simulink model "TestSolidStateTransformer"  (R2025b)
settings: Solver=VariableStepAuto  StartTime=0.0  StopTime=0.5  FixedStep=50e-6  RelTol=1e-3
model workspace (MAT data in the model file):
  sst.chb.Kbal = 0.000227272727273
  sst.dab.kp = 5.5
  sst.dab.ki = 130
  sst.dab.upperLimit = 0.45
  sst.dab.lowerLimit = -0.45
  sst.dab.sampleTime = 5e-05
  sst.dab.Kp_bal = 0.0005
  sst.dab.bal_alpha = 0.998116819821
  ups.sampleTime = 5e-05
undefined symbols (not defined in the file): DiscIntNeverNeededParam, ee_sli_rtmsupport, gcbh, Ts
libraries: fl_lib x23, nesl_utility x20, datacenter_lib x12, ee_lib x9, simulink x8, eeGeneralControl x6, eeTransforms x4, slpidlib x3, eeSinusoidalMeasurementV2 x2, simulink_extras x1
(part 1 of 2)
settings Model: SimulationMode=accelerator  Creator=saprasad  LastModifiedBy=skota
settings SimscapeCC: ExplicitSolverDiagnosticOptions=none

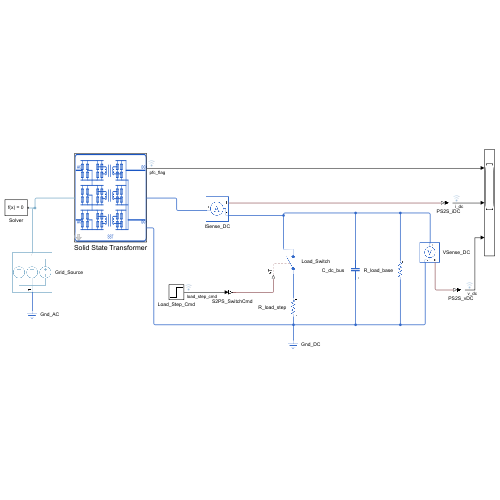
[thumbnail: Simulink's stored preview of the top-level diagram]
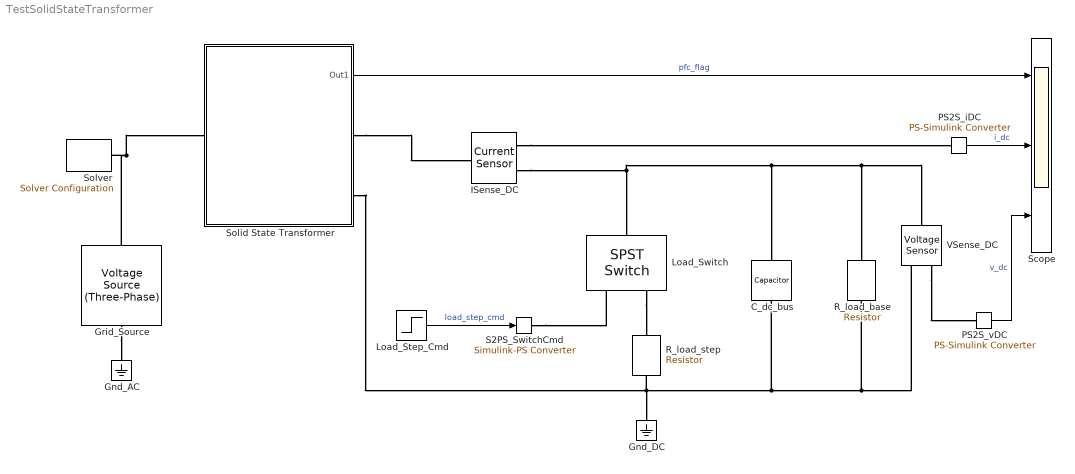
== system TestSolidStateTransformer ==
  C_dc_bus : ee_lib/Passive/Capacitor  cap_option=ee.enum.passive.capacitor.capOption.const  c=20e-3 F  Cvec=[1e-05, 1e-06] F  Vvec=[0, 10] V  CV_table_symmetry=ee.enum.passive.capacitor.tableSymmetry.yes  f_vec=[1, 10] kHz  DFext_vec=[.8, 1.2]  enable_C_tol=ee.enum.toleranceApplication.none  averaging_period=0 s  C_tol=5  tol_distribution=ee.enum.toleranceDistribution.uniform  nSigma=4  r=0 Ohm  g=0 1/Ohm  enable_operating_limits=ee.enum.enable.no  operating_limit_action=ee.enum.passive.reportOpLim.warn  max_working_voltage_range=[-25, 25] V  power_rating=1 W  maxTemperature=85 degC  thermalEnable=false  thermalMass=1 J/K  i_specify=off  i_priority=None  i=0 A  i_nominal_specify=off  i_nominal_value=1  i_nominal_unit=A  v_specify=off  v_priority=None  v=0 V  v_nominal_specify=off  v_nominal_value=1  v_nominal_unit=V  vc_specify=on  vc_priority=None  vc=800 V  vc_nominal_specify=off  vc_nominal_value=1  vc_nominal_unit=V  T_specify=off  T_priority=None  T=298.15 K  T_nominal_specify=off  T_nominal_value=1  T_nominal_unit=K
  Gnd_AC : fl_lib/Electrical/Electrical Elements/Electrical Reference
  Gnd_DC : fl_lib/Electrical/Electrical Elements/Electrical Reference
  Grid_Source : ee_lib/Sources/Voltage Source (Three-Phase)  vline_rms=13800 V  shift=0 deg  freq=60 Hz  impedance_option=1  SShortCircuit=1e9 A*V  XR=15  R=0.01 Ohm  L=3.97e-4 H  harmonic_option=0  harmonic_orders=[5, 7, 11, 13]  harmonic_ratios=[.1, .1, .1, .1]  G_parasitic=0 1/Ohm  I_specify=off  I_priority=None  I=[0, 0, 0] A  I_nominal_specify=off  I_nominal_value=1  I_nominal_unit=A
  ISense_DC : fl_lib/Electrical/Electrical Sensors/Current Sensor
  Load_Step_Cmd : Step  Time=0.3  SampleTime=0
  Load_Switch : ee_lib/Switches & Breakers/SPST Switch  R_closed=1e-3 Ohm  G_open=1e-8 S  Threshold=0.5 V  Width=0 V  model_dynamics=0  t_on=1e-3 s  t_off=1e-3 s  initial_vT=0 V
      settings: InternalSimscapePortConfiguration="{\"Bottom\":[],\"Left\":[{\"id\":\"vT\",\"label\":\"vT\",\"type\":\"input\"},{\"id\":\"p\",\"label\":\"\",\"type\":\"foundation.electrical.electrical\"}],\"Right\":[{\"id\":\"n\",\"label\":\"\",\"type\":\"foundation.electrical.electrical\"}],\"Top\":[]}"
  PS2S_iDC : nesl_utility/PS-Simulink Converter  PhysicalDomain=network_engine_domain  SubClassName=ps_output  LeftPortType=input  RightPortType=output  PseudoPeriodic=off  Frequencies=[]  VectorFormat=inherit  Unit=A  AffineConversion=off
  PS2S_vDC : nesl_utility/PS-Simulink Converter  PhysicalDomain=network_engine_domain  SubClassName=ps_output  LeftPortType=input  RightPortType=output  PseudoPeriodic=off  Frequencies=[]  VectorFormat=inherit  Unit=V  AffineConversion=off
  R_load_base : ee_lib/Passive/Resistor  R=0.32 Ohm  enable_R_tol=ee.enum.toleranceApplication.none  R_tol=5  tol_distribution=ee.enum.toleranceDistribution.uniform  nSigma=4  enable_operating_limits=ee.enum.enable.no  operating_limit_action=ee.enum.passive.reportOpLim.warn  power_rating=1 W  max_working_voltage=100 V  noise_mode=ee.enum.sources.noise.Disabled  Tdevice=25 degC  sample_time=1e-3 s  repeatability=ee.enum.ic.repeatability.notRepeatable  user_seed=0  auto_seed=2446450362  power_derating_T1=70 degC  power_derating_T2=155 degC  operating_temperature_range_vec=[-50, 150] degC  alpha=3.93e-3 1/K  Tmeas=25 degC  thermal_mass=100 J/K  temperature_specify=off  temperature_priority=High  temperature=298.15 K  temperature_nominal_specify=off  temperature_nominal_value=1  temperature_nominal_unit=K
  R_load_step : ee_lib/Passive/Resistor  R=0.32 Ohm  enable_R_tol=ee.enum.toleranceApplication.none  R_tol=5  tol_distribution=ee.enum.toleranceDistribution.uniform  nSigma=4  enable_operating_limits=ee.enum.enable.no  operating_limit_action=ee.enum.passive.reportOpLim.warn  power_rating=1 W  max_working_voltage=100 V  noise_mode=ee.enum.sources.noise.Disabled  Tdevice=25 degC  sample_time=1e-3 s  repeatability=ee.enum.ic.repeatability.notRepeatable  user_seed=0  auto_seed=3822851528  power_derating_T1=70 degC  power_derating_T2=155 degC  operating_temperature_range_vec=[-50, 150] degC  alpha=3.93e-3 1/K  Tmeas=25 degC  thermal_mass=100 J/K  temperature_specify=off  temperature_priority=High  temperature=298.15 K  temperature_nominal_specify=off  temperature_nominal_value=1  temperature_nominal_unit=K
  S2PS_SwitchCmd : nesl_utility/Simulink-PS Converter  PhysicalDomain=network_engine_domain  SubClassName=ps_input  LeftPortType=input  RightPortType=output  PseudoPeriodic=off  Frequencies=[]  NoiseDistribution=none  NoiseParameters=[]  Unit=1  AffineConversion=off  FilteringAndDerivatives=provide  SimscapeFilterOrder=1  InputFilterTimeConstant=0.001  UdotUserProvided=0
  Scope : Scope  NumInputPorts=3
      settings: ActiveDisplayYMinimum=-0.12499999999999997  ActiveDisplayYMaximum=1.125
  Solid State Transformer : Subsystem  mask(Solid State Transformer){inputVoltage=13800, dcBusVoltage=4400, dcOutputVoltage=800, frequency=60, numModules=3, Kp_dab=5.5, Ki_dab=130, dab_sat_upper=0.45, dab_sat_lower=-0.45, dcBusCapacitance=5e-3, filterInductance=10e-3, filterResistance=0.1, dab_sampleTime=50e-6, Vdc_init=4400}
      mask prompts: inputVoltage "Input Voltage - Phase to Phase RMS (V)"; dcBusVoltage "DC Bus Voltage per Module (V)"; dcOutputVoltage "DC Output Voltage (V)"; frequency "Grid Frequency (Hz)"; numModules "Number of CHB Modules per Phase"; Kp_dab "Proportional Gain (Kp)"; Ki_dab "Integral Gain (Ki)"; dab_sat_upper "Phase Shift Upper Limit"; dab_sat_lower "Phase Shift Lower Limit"; dcBusCapacitance "DC Bus Capacitance (F)"; filterInductance "Filter Inductance (H)"; filterResistance "Filter Resistance (Ohm)"; dab_sampleTime "DAB sample time (s)"; Vdc_init "Initial DC bus voltage (V)"
      mask help: Solid State Transformer with CHB rectifier and DAB DC-DC converters. Three-phase input, isolated DC output.
      mask init:
      | % SST Mask Initialization
      | % Propagate DAB PI gains to all 9 DAB controllers
      | phases = {'Subsystem1', 'Subsystem2', 'Subsystem3'};
      | 
      | % Support per-phase capacitance: scalar or [Ca Cb Cc] vector
      | if isscalar(dcBusCapacitance)
      |     capPerPhase = dcBusCapacitance * [1 1 1];
      | else
      |     capPerPhase = dcBusCapacitance;
      | end
      | 
      | % Support per-phase initial voltage: scalar or [Va Vb Vc] vector
      | if isscalar(Vdc_init)
      |     vInitPerPhase = Vdc_init * [1 1 1];
      | else
      |     vInitPerPhase = Vdc_init;
      | end
      | 
      | for p = 1:3
      |     % Propagate DC bus capacitance (per-phase)
      |     caps = {'Capacitor', 'Capacitor1', 'Capacitor2'};
      |     for c = 1:3
      |         capPath = [gcb, '/Converters/', phases{p}, '/', caps{c}];
      |         set_param(capPath, 'c', num2str(capPerPhase(p)));
      |         set_param(capPath, 'vc', num2str(vInitPerPhase(p)));
      |     end
      | end
      | 
      | % Propagate filter parameters
      | rlPath = [gcb, '/Filter & AC measurements/RL filter'];
      | set_param(rlPath, 'L', num2str(filterInductance));
      | set_param(rlPath, 'R', num2str(filterResistance));
      settings: CopyFcn=set_param(gcbh,'LinkStatus','none');
      mask Help: web("DocumentationSolidStateTransformer.html")
      mask DialogControl GeneralTab Prompt: General
      mask DialogControl PFCControlTab Prompt: PFC Control
      mask DialogControl openPFCController Prompt: Edit PFC Controller
      mask DialogControl openPFCController Callback:
      | blockPath = [gcb,'/PFC Rectifier Controller'];
      | open_system(blockPath, 'mask');
      mask DialogControl HBridgeTab Prompt: H-Bridge
      mask DialogControl openCHBBlock Prompt: Edit CHB Phase Leg Parameters
      mask DialogControl openCHBBlock Callback:
      | blockPath = [gcb,'/Converters/Subsystem1/CHB Phase Leg' char(10) '(Average Model)'];
      | open_system(blockPath, 'mask');
      mask DialogControl DABTab Prompt: DAB
      mask DialogControl openDABBlock Prompt: Edit DAB Parameters
      mask DialogControl openDABBlock Callback:
      | blockPath = [gcb,'/Converters/Subsystem1/DAB Generalized' char(10) 'Average Model'];
      | open_system(blockPath, 'mask');
      mask Display: image('sst_icon.svg')
  Solver : nesl_utility/Solver Configuration  PhysicalDomain=network_engine_domain  SubClassName=solver  LeftPortType=input  RightPortType=generic  Tones=[]  Harmonics=[]  SimulateNoise=off  Profile=off  UseLocalSampling=off  EnableSwitchedLinearOptims=on  FrequencyDomain=off  UseCCode=off  RelTol=0.001  AbsTol=0.001  MinStep=1e-09  ToWorkspace=off  RevertToSquareIcSolve=off  NumHomotopyIterations=100  PhasorMode=off  PhasorModeNumHarmonics=1  ConsistencySolver=NEWTON_XTOL_AFTER_FTOL  IndexReductionMethod=DerivativeReplacement  DoDC=off  ResidualTolerance=1e-09  ConsistencyTolSource=GLOBAL  ConsistencyAbsTol=0.001  ConsistencyRelTol=0.001  ConsistencyTolFactor=0.001  UseLocalSolver=on  LocalSolverChoice=NE_BACKWARD_EULER_ADVANCER  ResolveIndetEquations=off  FunctionEvalNumThread=1  LocalSolverSampleTime=5e-5  DoFixedCost=off  MaxNonlinIter=3  MaxModeIter=2  ComputeImpulses=off  ImpulseIterations=2  LinearAlgebra=auto  LinearAlgebraNumThread=0  EquationFormulation=NE_TIME_EF  DelaysMemoryBudget=1024  AutomaticFiltering=off  FilteringTimeConstant=0.001  PartitionStorageMethod=AS_NEEDED  PartitionMemoryBudget=1024  PartitionMethod=ROBUST  MultibodyUseLocalSolver=off  MultibodyLocalSolverChoice=ODE1  MultibodyLocalSolverSampleTime=0.001
  VSense_DC : fl_lib/Electrical/Electrical Sensors/Voltage Sensor
  wires:
  Solid State Transformer/1(Out1) -> Scope/1  "pfc_flag"
  Load_Step_Cmd/1 -> S2PS_SwitchCmd/1  "load_step_cmd"
  PS2S_iDC/1 -> Scope/2  "i_dc"
  PS2S_vDC/1 -> Scope/3  "v_dc"
  connections:
  Grid_Source/RConn1 -- Solid State Transformer/LConn1 -- Solver/RConn1
  Grid_Source/LConn1 -- Gnd_AC/LConn1
  Solid State Transformer/RConn1 -- ISense_DC/LConn1
  ISense_DC/RConn2 -- VSense_DC/LConn1 -- R_load_base/LConn1 -- C_dc_bus/LConn1 -- Load_Switch/RConn1
  Load_Switch/LConn2 -- R_load_step/LConn1
  Solid State Transformer/RConn2 -- VSense_DC/RConn2 -- R_load_base/RConn1 -- C_dc_bus/RConn1 -- Gnd_DC/LConn1 -- R_load_step/RConn1
  VSense_DC/RConn1 -- PS2S_vDC/LConn1
  ISense_DC/RConn1 -- PS2S_iDC/LConn1
  S2PS_SwitchCmd/RConn1 -- Load_Switch/LConn1

== system TestSolidStateTransformer/Solid State Transformer ==
  note: Rectifier Control
  note: DAB Control
  note: Cascaded H-Bridge modules with DAB
  Constant1 : Constant  Value=dcBusVoltage
  Constant2 : Constant  Value=0
  Converters : Subsystem
      settings: PortSchema="{\"entries\":[{\"content\":{\"sides\":[{\"content\":{\"connectorIds\":[\"In1\",\"In2\",\"LConn1\"]},\"type\":\"ConnectorPlacement.EquallySpacedRectSide\",\"uuid\":\"3c50ecae-d327-4517-ac35-d4ccad8214d6\"},{\"content\":{\"connectorIds\":[\"RConn1\",\"RConn2\",\"Out1\",\"Out2\"],\"side\":\"RIGHT\"},\"type\":\"ConnectorPlacement.EquallySpacedRectSide\",\"uuid\":\"ce483151-8cc4-4e89-a036-44eb982feae5\"},{\"content\":{\"side\":\"TOP\"},\"type\":\"ConnectorPlacement.EquallySpacedRectSide\",\"uuid\":\"39146706-ffb9-4bd3-97cb-72551c78d2ac\"}]},\"type\":\"ConnectorPlacement.EquallySpacedConnector\",\"uuid\":\"8cf16702-94fc-4b9b-91c9-b502d0239b3b\"}],\"packageUris\":[\"http://schema.mathworks.com/mf0/Connector/R2020b\"],\"version\":\"1.0\"}"
  DAB Controller : Subsystem
  DC Voltage Balancing : Subsystem
  Filter & AC measurements : Subsystem
  PFC Rectifier Controller : Subsystem  LoadFcn=%ee_sli_rtmsupport( 'loadfcn', gcbh );  mask(PFC Rectifier Controller (Three-Phase)){Freq=60, L=0.01, BaseImpedance=9.522, KpPLL=15, KiPLL=100, Ts=5e-05, KpVoltage=18, KiVoltage=500, KdVoltage=0, NdVoltage=100, BaseVdc=4400, VoltControlUpperLimit=1, VoltControlLowerLimit=-1, KpdCurrent=10, KidCurrent=200, KddCurrent=0, IdControlUpperLimit=1, IdControlLowerLimit=-1, KpqCurrent=10, KiqCurrent=200, KdqCurrent=0, NdCurrent=100, IqControlUpperLimit=1, IqControlLowerLimit=-1}
      mask prompts: Freq "physmod:ee:library:comments:control:eeConverterControllers:SystemFrequencyHz_MP"; L "physmod:ee:library:comments:control:eeConverterControllers:ACFilterInductanceH_MP"; BaseImpedance "physmod:ee:library:comments:control:eeConverterControllers:ACSideBaseImpedanceOhm_MP"; KpPLL "physmod:ee:library:comments:control:eeConverterControllers:PLLProportionalGain_MP"; KiPLL "physmod:ee:library:comments:control:eeConverterControllers:PLLIntegralGain_MP"; Ts "physmod:ee:library:comments:control:eeConverterControllers:SampleTime1ForInherited_MP"; KpVoltage "physmod:ee:library:comments:control:eeConverterControllers:ProportionalGain_MP"; KiVoltage "physmod:ee:library:comments:control:eeConverterControllers:IntegralGain_MP"; KdVoltage "physmod:ee:library:comments:control:eeConverterControllers:DerivativeGain_MP"; NdVoltage "physmod:ee:library:comments:control:eeConverterControllers:DerivativeControllerFilterCoefficientN_MP"; BaseVdc "physmod:ee:library:comments:control:eeConverterControllers:DCBusBaseVoltageV_MP"; VoltControlUpperLimit "physmod:ee:library:comments:control:eeConverterControllers:ControllerOutputUpperLimitpu_MP"; VoltControlLowerLimit "physmod:ee:library:comments:control:eeConverterControllers:ControllerOutputLowerLimitpu_MP"; KpdCurrent "physmod:ee:library:comments:control:eeConverterControllers:IdProportionalGain_MP"; KidCurrent "physmod:ee:library:comments:control:eeConverterControllers:IdIntegralGain_MP"; KddCurrent "physmod:ee:library:comments:control:eeConverterControllers:IdDerivativeGain_MP"; IdControlUpperLimit "physmod:ee:library:comments:control:eeConverterControllers:IdControllerOutputUpperLimitpu_MP"; IdControlLowerLimit "physmod:ee:library:comments:control:eeConverterControllers:IdControllerOutputLowerLimitpu_MP"; KpqCurrent "physmod:ee:library:comments:control:eeConverterControllers:IqProportionalGain_MP"; KiqCurrent "physmod:ee:library:comments:control:eeConverterControllers:IqIntegralGain_MP"; KdqCurrent "physmod:ee:library:comments:control:eeConverterControllers:IqDerivativeGain_MP"; NdCurrent "physmod:ee:library:comments:control:eeConverterControllers:DerivativeCurrentControllerFilterCoefficientN_MP"; IqControlUpperLimit "physmod:ee:library:comments:control:eeConverterControllers:IqControllerOutputUpperLimitpu_MP"; IqControlLowerLimit "physmod:ee:library:comments:control:eeConverterControllers:IqControllerOutputLowerLimitpu_MP"
      mask help: physmod:ee:library:comments:control:eeConverterControllers:PFCRectifierController_MD
      mask init:
      | ee.mask.initializePFCController(gcb,Ts, Freq, L,BaseImpedance,KpPLL,KiPLL,KpVoltage,KiVoltage,KdVoltage,BaseVdc, NdVoltage,VoltControlUpperLimit,VoltControlLowerLimit,KpdCurrent, KidCurrent, KddCurrent, NdCurrent, IdControlUpperLimit, IdControlLowerLimit, KpqCurrent, KiqCurrent, KdqCurrent, IqControlUpperLimit, IqControlLowerLimit);
      settings: CopyFcn=%ee_sli_rtmsupport( 'copyfcn', gcbh );  DeleteFcn=ee_sli_rtmsupport( 'deletefcn', gcbh );  ModelCloseFcn=ee_sli_rtmsupport( 'modelclosefcn', gcbh );  PostSaveFcn=ee_sli_rtmsupport( 'postsavefcn', gcbh );  PreCopyFcn=ee_sli_rtmsupport( 'precopyfcn', gcbh );  OpenFcn=ee_sli_rtmsupport( 'openfcn', gcbh );  CloseFcn=%ee_sli_rtmsupport( 'closefcn', gcbh );  PreDeleteFcn=ee_sli_rtmsupport( 'predeletefcn', gcbh );
      mask Help: web(nesl_help(gcbh))
      mask DialogControl GeneralTabVal Prompt: physmod:ee:library:comments:control:eeConverterControllers:tab_General
      mask DialogControl Freq Prompt: System frequency (Hz)
      mask DialogControl L Prompt: AC filter inductance (H)
      mask DialogControl BaseImpedance Prompt: AC side base impedance (Ohm)
      mask DialogControl KpPLL Prompt: PLL proportional gain
      mask DialogControl KiPLL Prompt: PLL integral gain
      mask DialogControl Ts Prompt: Sample time (-1 for inherited)
      mask DialogControl VoltageControl Prompt: physmod:ee:library:comments:control:eeConverterControllers:tab_VoltageController
      mask DialogControl KpVoltage Prompt: Proportional gain
      mask DialogControl KiVoltage Prompt: Integral gain
      mask DialogControl KdVoltage Prompt: Derivative gain
      mask DialogControl NdVoltage Prompt: Derivative controller filter coefficient (N)
      mask DialogControl BaseVdc Prompt: DC bus base voltage (V)
      mask DialogControl VoltControlUpperLimit Prompt: Controller output upper limit (pu)
      mask DialogControl VoltControlLowerLimit Prompt: Controller output lower limit (pu)
      mask DialogControl CurrentControl Prompt: physmod:ee:library:comments:control:eeConverterControllers:tab_CurrentController
      mask DialogControl KpdCurrent Prompt: Id proportional gain
      mask DialogControl KidCurrent Prompt: Id integral gain
      mask DialogControl KddCurrent Prompt: Id derivative gain
      mask DialogControl IdControlUpperLimit Prompt: Id controller output upper limit (pu)
      mask DialogControl IdControlLowerLimit Prompt: Id controller output lower limit (pu)
      mask DialogControl KpqCurrent Prompt: Iq proportional gain
      mask DialogControl KiqCurrent Prompt: Iq integral gain
      mask DialogControl KdqCurrent Prompt: Iq derivative gain
      mask DialogControl NdCurrent Prompt: Derivative current controller filter coefficient (N)
      mask DialogControl IqControlUpperLimit Prompt: Iq controller output upper limit (pu)
      mask DialogControl IqControlLowerLimit Prompt: Iq controller output lower limit (pu)
  + : PMIOPort  Side=Right
  - : PMIOPort  Port=2  Side=Right
  ABC : PMIOPort  Port=3  Side=Left
  Out1 : Outport
  wires:
  PFC Rectifier Controller/3(Flag) -> Out1/1
  PFC Rectifier Controller/2(Visualization) -> DAB Controller/2(Vac)
  PFC Rectifier Controller/1(VabcRef (pu)) -> DC Voltage Balancing/2(VabcRef)
  DAB Controller/1(phi) -> Converters/2(phi)
  Converters/1(Vdc) -> DC Voltage Balancing/1(Vdc), DAB Controller/1(Vdc)
  DC Voltage Balancing/1(mabc) -> Converters/1(mabc)
  Filter & AC measurements/2(Iabc) -> PFC Rectifier Controller/5(IabcSens (pu))
  Converters/2(VdcMeas) -> PFC Rectifier Controller/3(VdcSens (V))
  Filter & AC measurements/1(Vabc) -> PFC Rectifier Controller/4(VabcSens (pu))
  Constant1/1 -> PFC Rectifier Controller/1(VdcRef (V))
  Constant2/1 -> PFC Rectifier Controller/2(QRef (pu))
  connections:
  Filter & AC measurements/RConn1 -- Converters/LConn1
  +/RConn1 -- Converters/RConn1
  -/RConn1 -- Converters/RConn2
  Filter & AC measurements/LConn1 -- ABC/RConn1

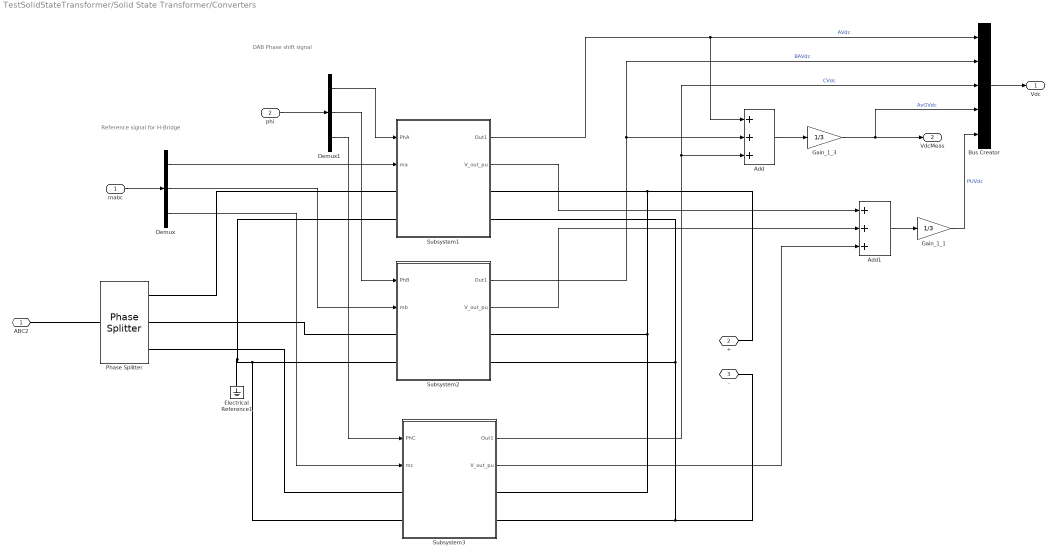
== system TestSolidStateTransformer/Solid State Transformer/Converters ==
  note: Reference signal for H-Bridge
  note: DAB Phase shift signal
  mabc : Inport
  phi : Inport  Port=2
  Add : Sum  Inputs=+++
  Add1 : Sum  Inputs=+++
  Bus Creator : BusCreator  Inputs=5
  Demux : Demux  Outputs=3
  Demux1 : Demux  Outputs=3
  Electrical Reference1 : fl_lib/Electrical/Electrical Elements/Electrical Reference
  Gain_1_1 : Gain  Gain=1/3
  Gain_1_3 : Gain  Gain=1/3
  Phase Splitter : ee_lib/Connectors & References/Phase Splitter
  Subsystem1 : Subsystem
  Subsystem2 : Subsystem
  Subsystem3 : Subsystem
  ABC2 : PMIOPort  Side=Left
  + : PMIOPort  Port=2  Side=Right
  - : PMIOPort  Port=3  Side=Right
  Vdc : Outport
  VdcMeas : Outport  Port=2
  wires:
  Demux/3 -> Subsystem3/2(mc)
  Demux/2 -> Subsystem2/2(mb)
  Demux/1 -> Subsystem1/2(ma)
  mabc/1 -> Demux/1
  Demux1/3 -> Subsystem3/1(PhC)
  Demux1/2 -> Subsystem2/1(PhB)
  Demux1/1 -> Subsystem1/1(PhA)
  Gain_1_1/1 -> Bus Creator/5  "PUVdc"
  Add1/1 -> Gain_1_1/1
  Subsystem3/2(V_out_pu) -> Add1/3
  Subsystem1/2(V_out_pu) -> Add1/1
  Subsystem2/2(V_out_pu) -> Add1/2
  phi/1 -> Demux1/1
  Bus Creator/1 -> Vdc/1
  Gain_1_3/1 -> Bus Creator/4, VdcMeas/1  "AvGVdc"
  Add/1 -> Gain_1_3/1
  Subsystem3/1(Out1) -> Add/3, Bus Creator/3  "CVdc"
  Subsystem2/1(Out1) -> Bus Creator/2, Add/2  "BAVdc"
  Subsystem1/1(Out1) -> Add/1, Bus Creator/1  "AVdc"
  connections:
  Phase Splitter/LConn1 -- ABC2/RConn1
  +/RConn1 -- Subsystem2/RConn1 -- Subsystem3/RConn1 -- Subsystem1/RConn1
  Subsystem2/LConn1 -- Phase Splitter/RConn2
  Subsystem2/RConn2 -- -/RConn1 -- Subsystem3/RConn2 -- Subsystem1/RConn2
  Subsystem1/LConn1 -- Phase Splitter/RConn1
  Subsystem3/LConn1 -- Phase Splitter/RConn3
  Electrical Reference1/LConn1 -- Subsystem3/LConn2 -- Subsystem2/LConn2 -- Subsystem1/LConn2

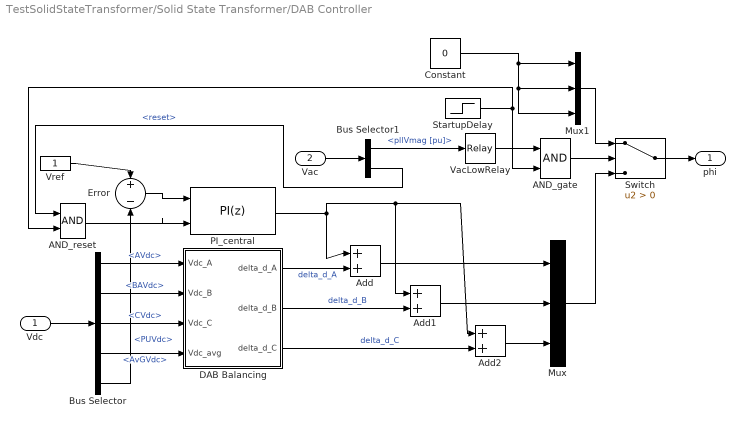
== system TestSolidStateTransformer/Solid State Transformer/DAB Controller ==
  Vdc : Inport
  Vac : Inport  Port=2
  AND_gate : Logic  AllPortsSameDT=off  OutDataTypeStr=boolean
  AND_reset : Logic  AllPortsSameDT=off  OutDataTypeStr=boolean
  Add : Sum
  Add1 : Sum
  Add2 : Sum
  Bus Selector : BusSelector  OutputSignals=AVdc,BAVdc,CVdc,AvGVdc,PUVdc
  Bus Selector1 : BusSelector  OutputSignals=pllVmag [pu],reset
  Constant : Constant  Value=0
  DAB Balancing : Subsystem
  Error : Sum  Inputs=+-
  Mux : Mux  Inputs=3
  Mux1 : Mux  Inputs=3
  PI_central : slpidlib/PID Controller  Controller=PI  Form=Parallel  TimeDomain=Discrete-time  UseExternalTs=off  SampleTime=5e-05  IntegratorMethod=Forward Euler  FilterMethod=Forward Euler  ControllerParametersSource=internal  P=5.5  I=130  UseKiTs=off  D=0  UseExternalDerivativeSource=off  N=100  UseFilter=on  TunerSelectOption=Transfer Function Based (PID Tuner App)  InitialConditionSource=internal  InitialConditionForIntegrator=0  InitialConditionForFilter=0  DifferentiatorICPrevScaledInput=0  ExternalReset=falling  TrackingMode=off  Kt=1  LimitOutput=on  SatLimitsSource=internal  UpperSaturationLimit=0.45  LowerSaturationLimit=-0.45  LinearizeAsGain=off  AntiWindupMode=none  Kb=1  LimitIntegrator=off  UpperIntegratorSaturationLimit=inf  LowerIntegratorSaturationLimit=-inf  POutMin=[]  POutMax=[]  IOutMin=[]  IOutMax=[]  DOutMin=[]  DOutMax=[]  NOutMin=[]  NOutMax=[]  SumOutMin=[]  SumOutMax=[]  SaturationOutMin=[]  SaturationOutMax=[]  PParamMin=[]  PParamMax=[]  IParamMin=[]  IParamMax=[]  DParamMin=[]  DParamMax=[]  NParamMin=[]  NParamMax=[]  KbParamMin=[]  KbParamMax=[]  KtParamMin=[]  KtParamMax=[]  KbOutMin=[]  KbOutMax=[]  KtOutMin=[]  KtOutMax=[]  IntegratorOutMin=[]  IntegratorOutMax=[]  FilterOutMin=[]  FilterOutMax=[]  SumI1OutMin=[]  SumI1OutMax=[]  SumI2OutMin=[]  SumI2OutMax=[]  SumI3OutMin=[]  SumI3OutMax=[]  SumI4OutMin=[]  SumI4OutMax=[]  SumDOutMin=[]  SumDOutMax=[]  DifferentiatorOutMin=[]  DifferentiatorOutMax=[]  FilterDiffOutCoefMin=[]  FilterDiffOutCoefMax=[]  ReciprocalOutMin=[]  ReciprocalOutMax=[]  SumDenOutMin=[]  SumDenOutMax=[]  SumNumOutMin=[]  SumNumOutMax=[]  DivideOutMin=[]  DivideOutMax=[]  UdiffTsProdOutMin=[]  UdiffTsProdOutMax=[]  NTsProdOutMin=[]  NTsProdOutMax=[]  UintegralTsProdOutMin=[]  UintegralTsProdOutMax=[]  UngainTsProdOutMin=[]  UngainTsProdOutMax=[]  ClampingZeroOutDataTypeStr=Inherit: Inherit via back propagation  ClampingZeroOutMin=[]  ClampingZeroOutMax=[]  FilterDenConstantOutDataTypeStr=Inherit: Inherit via back propagation  FilterDenConstantOutMin=[]  FilterDenConstantOutMax=[]  PCopyOutDataTypeStr=Inherit: Inherit via back propagation  PCopyOutMin=[]  PCopyOutMax=[]  NCopyOutDataTypeStr=Inherit: Inherit via back propagation  NCopyOutMin=[]  NCopyOutMax=[]  IntegratorContinuousStateAttributes=''  IntegratorStateMustResolveToSignalObject=off  IntegratorRTWStateStorageClass=Auto  FilterContinuousStateAttributes=''  FilterStateMustResolveToSignalObject=off  FilterRTWStateStorageClass=Auto  ParallelPVariant=InternalParameters  IdealPVariant=Disabled  IVariant=InternalParameters  DVariant=Disabled  IntegratorVariant=Discrete  SatVariant=Enabled  AWVariant=Passthrough  PCopyVariant=Disabled  TRVariant=Disabled  FdbkBlocksVariant=Forward  IdealPFdbkVariant=Disabled  SatFdbkVariant=Disabled  DerivativeFilterVariant=Disabled  NVariant=Disabled  NCopyVariant=Disabled_SignalSpec  FilterICVariant=Disabled  IntegratorICVariant=InternalICs  ExternalResetVariant=ExternalReset  TRSumVariant=Passthrough  SumFdbkVariant=Disabled  SumVariant=Sum_PI  TsampFilterVariant=InternalTs  TsampNgainVariant=Passthrough  TsampIntegralVariant=Disabled_SignalSpec  ExternalSaturationOutDataTypeStr=Inherit: Same as second input  DerivativeSourceVariant=Disabled  PreIntVariant=InternalPreInt
      settings: LibrarySourceBlock=simulink/Discrete/Discrete PID Controller
  StartupDelay : Step  SampleTime=0
  Switch : Switch  Criteria=u2 > Threshold  SaturateOnIntegerOverflow=off  InputSameDT=off
  VacLowRelay : Relay  OnSwitchValue=0.48  OffSwitchValue=0.42  OnOutputValue=0  OffOutputValue=1
  Vref : Constant
  phi : Outport
  wires:
  VacLowRelay/1 -> AND_gate/1
  AND_reset/1 -> PI_central/2
  Bus Selector1/2 -> AND_reset/1  "<reset>"
  AND_gate/1 -> Switch/2
  StartupDelay/1 -> AND_reset/2, AND_gate/2
  Mux1/1 -> Switch/1
  Constant/1 -> Mux1/1, Mux1/2, Mux1/3
  Switch/1 -> phi/1
  Bus Selector1/1 -> VacLowRelay/1  "<pllVmag [pu]>"
  Vac/1 -> Bus Selector1/1
  Mux/1 -> Switch/3
  Add1/1 -> Mux/2
  Add2/1 -> Mux/3
  Add/1 -> Mux/1
  DAB Balancing/3(delta_d_C) -> Add2/2  "delta_d_C"
  DAB Balancing/2(delta_d_B) -> Add1/2  "delta_d_B"
  DAB Balancing/1(delta_d_A) -> Add/2  "delta_d_A"
  Bus Selector/5 -> Error/2  "<PUVdc>"
  Bus Selector/4 -> DAB Balancing/4(Vdc_avg)  "<AvGVdc>"
  Bus Selector/3 -> DAB Balancing/3(Vdc_C)  "<CVdc>"
  Bus Selector/2 -> DAB Balancing/2(Vdc_B)  "<BAVdc>"
  Bus Selector/1 -> DAB Balancing/1(Vdc_A)  "<AVdc>"
  Vdc/1 -> Bus Selector/1
  PI_central/1 -> Add/1, Add2/1, Add1/1
  Error/1 -> PI_central/1
  Vref/1 -> Error/1

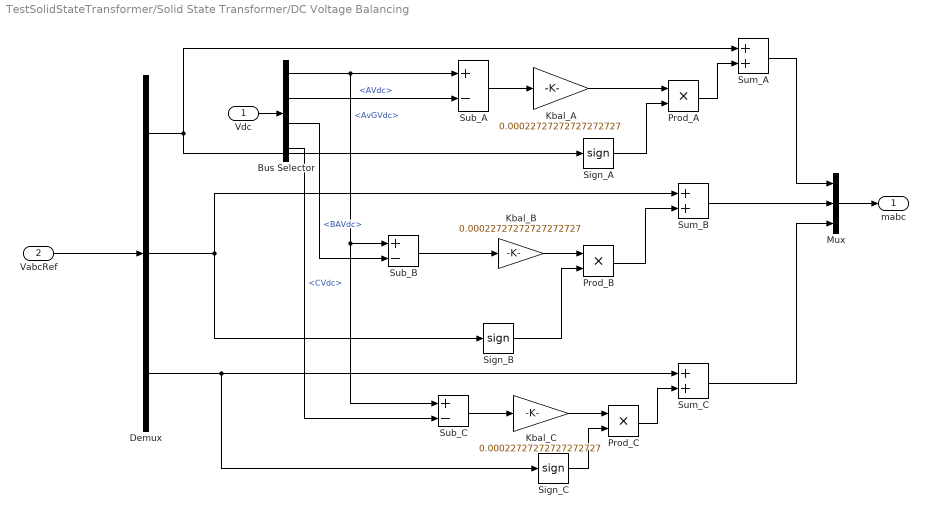
== system TestSolidStateTransformer/Solid State Transformer/DC Voltage Balancing ==
  Vdc : Inport
  VabcRef : Inport  Port=2
  Bus Selector : BusSelector  OutputSignals=AvGVdc,AVdc,BAVdc,CVdc
  Demux : Demux  Outputs=3
  Kbal_A : Gain  Gain=0.00022727272727272727
  Kbal_B : Gain  Gain=0.00022727272727272727
  Kbal_C : Gain  Gain=0.00022727272727272727
  Mux : Mux  Inputs=3
  Prod_A : Product
  Prod_B : Product
  Prod_C : Product
  Sign_A : Signum
  Sign_B : Signum
  Sign_C : Signum
  Sub_A : Sum  Inputs=+-
  Sub_B : Sum  Inputs=+-
  Sub_C : Sum  Inputs=+-
  Sum_A : Sum
  Sum_B : Sum
  Sum_C : Sum
  mabc : Outport
  wires:
  Bus Selector/4 -> Sub_C/2  "<CVdc>"
  Bus Selector/3 -> Sub_B/2  "<BAVdc>"
  Bus Selector/2 -> Sub_A/2  "<AVdc>"
  Vdc/1 -> Bus Selector/1
  Mux/1 -> mabc/1
  Sum_C/1 -> Mux/3
  Sum_A/1 -> Mux/1
  Sum_B/1 -> Mux/2
  Demux/3 -> Sum_C/1, Sign_C/1
  Demux/2 -> Sign_B/1, Sum_B/1
  Demux/1 -> Sign_A/1, Sum_A/1
  VabcRef/1 -> Demux/1
  Bus Selector/1 -> Sub_A/1, Sub_B/1, Sub_C/1  "<AvGVdc>"
  Prod_C/1 -> Sum_C/2
  Prod_A/1 -> Sum_A/2
  Sign_B/1 -> Prod_B/2
  Kbal_B/1 -> Prod_B/1
  Sign_C/1 -> Prod_C/2
  Kbal_C/1 -> Prod_C/1
  Sign_A/1 -> Prod_A/2
  Kbal_A/1 -> Prod_A/1
  Sub_C/1 -> Kbal_C/1
  Sub_A/1 -> Kbal_A/1
  Prod_B/1 -> Sum_B/2
  Sub_B/1 -> Kbal_B/1

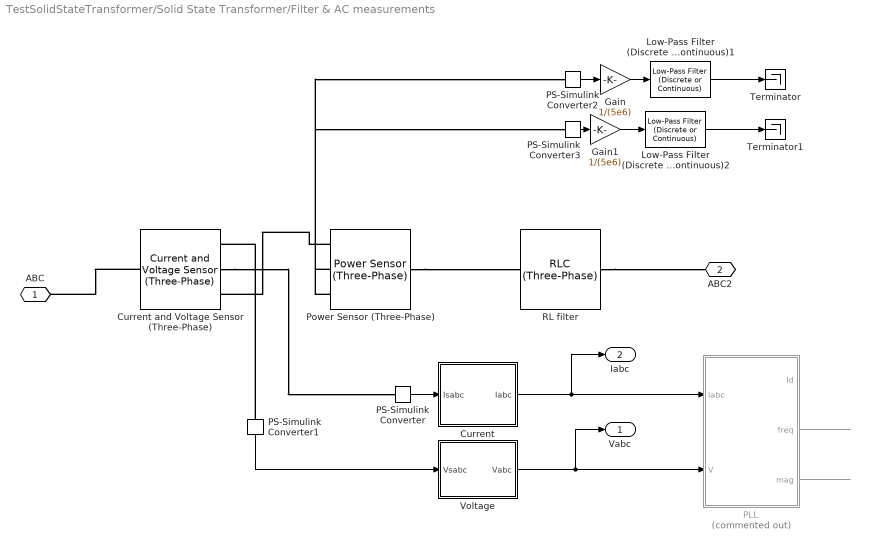
== system TestSolidStateTransformer/Solid State Transformer/Filter & AC measurements ==
  Current : Subsystem
  Current and Voltage Sensor (Three-Phase) : ee_lib/Sensors & Transducers/Current and Voltage Sensor (Three-Phase)  vMeasurementType=ee.enum.vmeasurement.lg  outputUnit=ee.enum.unit.pu  SRated=20e6 A*V  VRated=13800 V  I_specify=off  I_priority=None  I=[0, 0, 0] A  I_nominal_specify=off  I_nominal_value=1  I_nominal_unit=A  V_specify=off  V_priority=None  V=[0, 0, 0] V  V_nominal_specify=off  V_nominal_value=1  V_nominal_unit=V
      settings: InternalSimscapePortConfiguration="{\"Bottom\":[],\"Left\":[{\"id\":\"N1\",\"label\":\"~1\",\"type\":\"foundation.electrical.three_phase\"}],\"Right\":[{\"id\":\"V_output\",\"label\":\"V\",\"type\":\"output\"},{\"id\":\"I_output\",\"label\":\"I\",\"type\":\"output\"},{\"id\":\"N2\",\"label\":\"~2\",\"type\":\"foundation.electrical.three_phase\"}],\"Top\":[]}"
  Gain : Gain  Gain=1/(5e6)
  Gain1 : Gain  Gain=1/(5e6)
  Low-Pass Filter (Discrete or Continuous)1 : eeGeneralControl/Low-Pass Filter (Discrete or Continuous)  K=1  T=10e-3  B=inf  A=-inf  init_option=Inherited from block input  x0=0  Ts=-1
  Low-Pass Filter (Discrete or Continuous)2 : eeGeneralControl/Low-Pass Filter (Discrete or Continuous)  K=1  T=10e-3  B=inf  A=-inf  init_option=Inherited from block input  x0=0  Ts=-1
  PLL : Subsystem  Commented=on
      settings: PortSchema="{\"entries\":[{\"content\":{\"sides\":[{\"content\":{\"connectorIds\":[\"Out1\",\"Out2\",\"Out3\"]},\"type\":\"ConnectorPlacement.EquallySpacedRectSide\",\"uuid\":\"76485780-20fe-4fcf-8224-69648da6ed2a\"},{\"content\":{\"connectorIds\":[\"In1\",\"In2\"],\"side\":\"RIGHT\"},\"type\":\"ConnectorPlacement.EquallySpacedRectSide\",\"uuid\":\"f19a6390-e634-42c7-8d46-4cd80cbab182\"},{\"content\":{\"side\":\"TOP\"},\"type\":\"ConnectorPlacement.EquallySpacedRectSide\",\"uuid\":\"87682f72-1844-428e-be70-ad7ca3191ee3\"}]},\"type\":\"ConnectorPlacement.EquallySpacedConnector\",\"uuid\":\"f2136b07-48ec-402b-adb3-18c0bac2157c\"}],\"packageUris\":[\"http://schema.mathworks.com/mf0/Connector/R2020b\"],\"version\":\"1.0\"}"
  PS-Simulink Converter : nesl_utility/PS-Simulink Converter  PhysicalDomain=network_engine_domain  SubClassName=ps_output  LeftPortType=input  RightPortType=output  PseudoPeriodic=off  Frequencies=[]  VectorFormat=1-D array  Unit=inherit  AffineConversion=off
  PS-Simulink Converter1 : nesl_utility/PS-Simulink Converter  PhysicalDomain=network_engine_domain  SubClassName=ps_output  LeftPortType=input  RightPortType=output  PseudoPeriodic=off  Frequencies=[]  VectorFormat=1-D array  Unit=inherit  AffineConversion=off
  PS-Simulink Converter2 : nesl_utility/PS-Simulink Converter  PhysicalDomain=network_engine_domain  SubClassName=ps_output  LeftPortType=input  RightPortType=output  PseudoPeriodic=off  Frequencies=[]  VectorFormat=inherit  Unit=inherit  AffineConversion=off
  PS-Simulink Converter3 : nesl_utility/PS-Simulink Converter  PhysicalDomain=network_engine_domain  SubClassName=ps_output  LeftPortType=input  RightPortType=output  PseudoPeriodic=off  Frequencies=[]  VectorFormat=inherit  Unit=inherit  AffineConversion=off
  Power Sensor (Three-Phase) : ee_lib/Sensors & Transducers/Power Sensor (Three-Phase)  load_type=ee.enum.passive.type_balanced.balanced  f0=60 Hz
      settings: InternalSimscapePortConfiguration="{\"Bottom\":[],\"Left\":[{\"id\":\"N1\",\"label\":\"~1\",\"type\":\"foundation.electrical.three_phase\"}],\"Right\":[{\"id\":\"N2\",\"label\":\"~2\",\"type\":\"foundation.electrical.three_phase\"}],\"Top\":[{\"id\":\"Pm\",\"label\":\"P\",\"type\":\"output\"},{\"id\":\"Qm\",\"label\":\"Q\",\"type\":\"output\"}]}"
  RL filter : ee_lib/Passive/RLC Assemblies/RLC (Three-Phase)  port_option=ee.enum.threePhasePort.composite  component_structure=ee.enum.rlc.structure.SeriesRL  R=0.1 Ohm  L=0.01 H  C=1e-6 F  R_parasitic=1e-6 Ohm  G_parasitic=1e-6 1/Ohm  IL_specify=on  IL_priority=None  IL=[0, 0, 0] A  IL_nominal_specify=off  IL_nominal_value=1  IL_nominal_unit=A  VC_specify=on  VC_priority=None  VC=[0, 0, 0] V  VC_nominal_specify=off  VC_nominal_value=1  VC_nominal_unit=V
      settings: InternalSimscapePortConfiguration="{\"Bottom\":[],\"Left\":[{\"id\":\"N1\",\"label\":\"~1\",\"type\":\"foundation.electrical.three_phase\"}],\"Right\":[{\"id\":\"N2\",\"label\":\"~2\",\"type\":\"foundation.electrical.three_phase\"}],\"Top\":[]}"
  Terminator : Terminator
  Terminator1 : Terminator
  Voltage : Subsystem
  ABC : PMIOPort  Side=Left
  ABC2 : PMIOPort  Port=2  Side=Right
  Vabc : Outport
  Iabc : Outport  Port=2
  wires:
  Low-Pass Filter (Discrete or Continuous)2/1 -> Terminator1/1
  Low-Pass Filter (Discrete or Continuous)1/1 -> Terminator/1
  PLL/2(freq) -> ?
  PLL/3(mag) -> ?
  Gain1/1 -> Low-Pass Filter (Discrete or Continuous)2/1
  Gain/1 -> Low-Pass Filter (Discrete or Continuous)1/1
  PS-Simulink Converter3/1 -> Gain1/1
  PS-Simulink Converter2/1 -> Gain/1
  Voltage/1(Vabc) -> PLL/2(V), Vabc/1
  PS-Simulink Converter1/1 -> Voltage/1(Vsabc)
  Current/1(Iabc) -> PLL/1(Iabc), Iabc/1
  PS-Simulink Converter/1 -> Current/1(Isabc)
  connections:
  Power Sensor (Three-Phase)/LConn1 -- Current and Voltage Sensor (Three-Phase)/RConn3
  RL filter/RConn1 -- ABC2/RConn1
  Power Sensor (Three-Phase)/LConn3 -- PS-Simulink Converter3/LConn1
  Power Sensor (Three-Phase)/LConn2 -- PS-Simulink Converter2/LConn1
  Power Sensor (Three-Phase)/RConn1 -- RL filter/LConn1
  Current and Voltage Sensor (Three-Phase)/LConn1 -- ABC/RConn1
  PS-Simulink Converter1/LConn1 -- Current and Voltage Sensor (Three-Phase)/RConn1
  Current and Voltage Sensor (Three-Phase)/RConn2 -- PS-Simulink Converter/LConn1

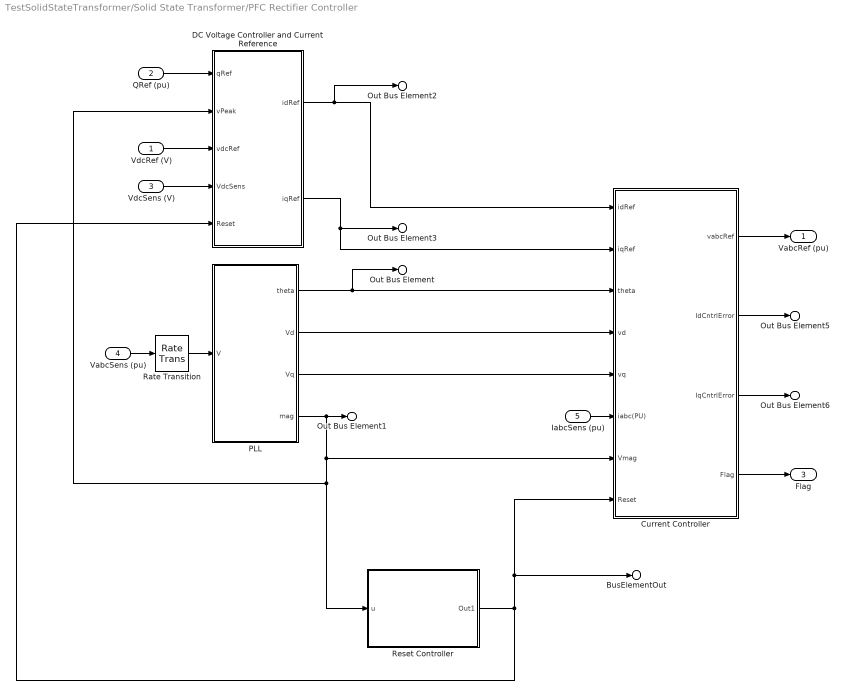
== system TestSolidStateTransformer/Solid State Transformer/PFC Rectifier Controller ==
  VdcRef (V) : Inport
  QRef (pu) : Inport  Port=2
  VdcSens (V) : Inport  Port=3
  VabcSens (pu) : Inport  Port=4
  IabcSens (pu) : Inport  Port=5
  Current Controller : Subsystem
  DC Voltage Controller and Current Reference : Subsystem
  PLL : Subsystem
      settings: PortSchema="{\"entries\":[{\"content\":{\"sides\":[{\"content\":{\"connectorIds\":[\"Out1\",\"Out2\",\"Out3\",\"Out4\"]},\"type\":\"ConnectorPlacement.EquallySpacedRectSide\",\"uuid\":\"76485780-20fe-4fcf-8224-69648da6ed2a\"},{\"content\":{\"connectorIds\":[\"In1\"],\"side\":\"RIGHT\"},\"type\":\"ConnectorPlacement.EquallySpacedRectSide\",\"uuid\":\"f19a6390-e634-42c7-8d46-4cd80cbab182\"},{\"content\":{\"side\":\"TOP\"},\"type\":\"ConnectorPlacement.EquallySpacedRectSide\",\"uuid\":\"87682f72-1844-428e-be70-ad7ca3191ee3\"}]},\"type\":\"ConnectorPlacement.EquallySpacedConnector\",\"uuid\":\"f2136b07-48ec-402b-adb3-18c0bac2157c\"}],\"packageUris\":[\"http://schema.mathworks.com/mf0/Connector/R2020b\"],\"version\":\"1.0\"}"
  Rate Transition : RateTransition  InitialCondition=1  OutPortSampleTime=Ts
  Reset Controller : Subsystem
  VabcRef (pu) : Outport
  Out Bus Element : Outport  Port=2  PortName=Visualization  Element=pllAngle [rad]
  Out Bus Element1 : Outport  Port=2  PortName=Visualization  Element=pllVmag [pu]
  Out Bus Element2 : Outport  Port=2  PortName=Visualization  Element=Idref [pu]
  Out Bus Element3 : Outport  Port=2  PortName=Visualization  Element=Iqref [pu]
  Out Bus Element5 : Outport  Port=2  PortName=Visualization  Element=IdCntrlError [pu]
  Out Bus Element6 : Outport  Port=2  PortName=Visualization  Element=IqCntrlError [pu]
  BusElementOut : Outport  Port=2  PortName=Visualization  Element=reset
  Flag : Outport  Port=3
  wires:
  Reset Controller/1(Out1) -> DC Voltage Controller and Current Reference/5(Reset), BusElementOut/1, Current Controller/8(Reset)
  Current Controller/4(Flag) -> Flag/1
  PLL/2(Vd) -> Current Controller/4(vd)
  VdcRef (V)/1 -> DC Voltage Controller and Current Reference/3(vdcRef)
  VabcSens (pu)/1 -> Rate Transition/1
  QRef (pu)/1 -> DC Voltage Controller and Current Reference/1(qRef)
  PLL/4(mag) -> Out Bus Element1/1, DC Voltage Controller and Current Reference/2(vPeak), Reset Controller/1(u), Current Controller/7(Vmag)
  Current Controller/1(vabcRef) -> VabcRef (pu)/1
  VdcSens (V)/1 -> DC Voltage Controller and Current Reference/4(VdcSens)
  PLL/3(Vq) -> Current Controller/5(vq)
  IabcSens (pu)/1 -> Current Controller/6(iabc(PU))
  DC Voltage Controller and Current Reference/1(idRef) -> Current Controller/1(idRef), Out Bus Element2/1
  DC Voltage Controller and Current Reference/2(iqRef) -> Out Bus Element3/1, Current Controller/2(iqRef)
  Rate Transition/1 -> PLL/1(V)
  PLL/1(theta) -> Current Controller/3(theta), Out Bus Element/1
  Current Controller/2(IdCntrlError) -> Out Bus Element5/1
  Current Controller/3(IqCntrlError) -> Out Bus Element6/1

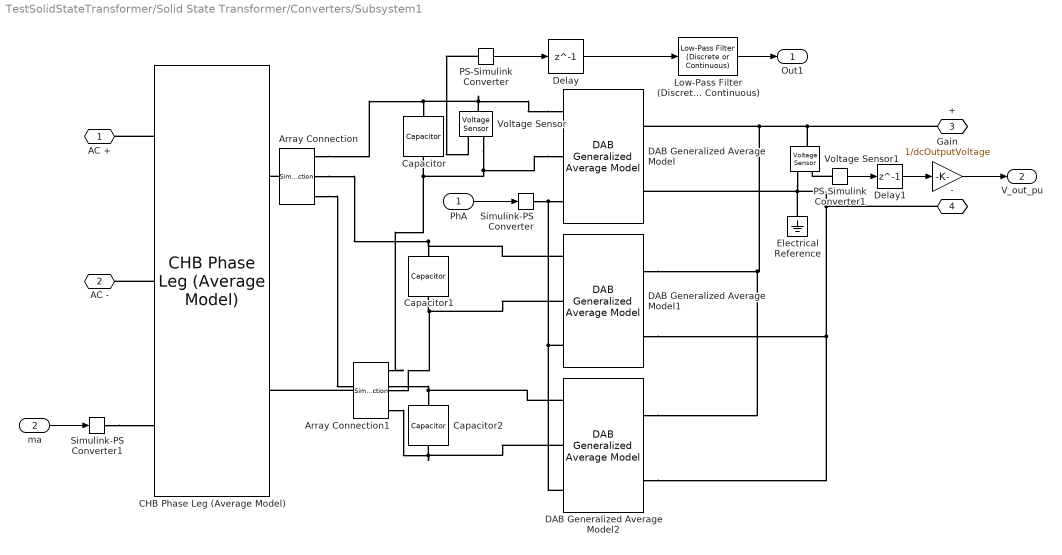
== system TestSolidStateTransformer/Solid State Transformer/Converters/Subsystem1 ==
  PhA : Inport
  ma : Inport  Port=2
  Array Connection : SimscapeArrayConnection  NumScalarElements=3
  Array Connection1 : SimscapeArrayConnection  NumScalarElements=3
  CHB Phase Leg (Average Model) : datacenter_lib/CHB Phase Leg (Average Model)  NumModules=3  OnResistance=1e-3 Ohm  InitialDCVoltage=4400 V  GridVoltage=13800 V  TotalDCVoltage=13200 V
      settings: InternalSimscapePortConfiguration="{\"Bottom\":[],\"Left\":[{\"id\":\"ACPositive\",\"label\":\"AC+\",\"type\":\"foundation.electrical.electrical\"},{\"id\":\"ACNegative\",\"label\":\"AC-\",\"type\":\"foundation.electrical.electrical\"},{\"id\":\"m\",\"label\":\"m\",\"type\":\"input\"}],\"Right\":[{\"id\":\"DCPositive\",\"label\":\"DC+\",\"type\":\"foundation.electrical.electrical\"},{\"id\":\"DCNegative\",\"label\":\"DC-\",\"type\":\"foundation.electrical.electrical\"}],\"Top\":[]}"
  Capacitor : fl_lib/Electrical/Electrical Elements/Capacitor  c=0.005 F  r=1e-6 Ohm  g=0 1/Ohm  i_specify=off  i_priority=None  i=0 A  i_nominal_specify=off  i_nominal_value=1  i_nominal_unit=A  v_specify=off  v_priority=None  v=0 V  v_nominal_specify=off  v_nominal_value=1  v_nominal_unit=V  vc_specify=on  vc_priority=None  vc=4400 V  vc_nominal_specify=off  vc_nominal_value=1  vc_nominal_unit=V
  Capacitor1 : fl_lib/Electrical/Electrical Elements/Capacitor  c=0.005 F  r=1e-6 Ohm  g=0 1/Ohm  i_specify=off  i_priority=None  i=0 A  i_nominal_specify=off  i_nominal_value=1  i_nominal_unit=A  v_specify=off  v_priority=None  v=0 V  v_nominal_specify=off  v_nominal_value=1  v_nominal_unit=V  vc_specify=on  vc_priority=None  vc=4400 V  vc_nominal_specify=off  vc_nominal_value=1  vc_nominal_unit=V
  Capacitor2 : fl_lib/Electrical/Electrical Elements/Capacitor  c=0.005 F  r=1e-6 Ohm  g=0 1/Ohm  i_specify=off  i_priority=None  i=0 A  i_nominal_specify=off  i_nominal_value=1  i_nominal_unit=A  v_specify=off  v_priority=None  v=0 V  v_nominal_specify=off  v_nominal_value=1  v_nominal_unit=V  vc_specify=on  vc_priority=None  vc=4400 V  vc_nominal_specify=off  vc_nominal_value=1  vc_nominal_unit=V
  DAB Generalized Average Model : datacenter_lib/DAB Generalized Average Model  N=5.5  L1=3.4e-05 H  L2=1.12e-06 H  Rt=0.005 Ohm  Co=0.001 F  fs=20000 Hz  vo0_init=800 V  it1R_init=0 A  it1I_init=0 A  include_esr=false  Rc=0.25 Ohm  i_in_specify=on  i_in_priority=None  i_in=0 A  i_in_nominal_specify=off  i_in_nominal_value=1  i_in_nominal_unit=A  i_out_specify=on  i_out_priority=None  i_out=0 A  i_out_nominal_specify=off  i_out_nominal_value=1  i_out_nominal_unit=A  v_in_specify=on  v_in_priority=None  v_in=0 V  v_in_nominal_specify=off  v_in_nominal_value=1  v_in_nominal_unit=V  v_out_specify=on  v_out_priority=None  v_out=0 V  v_out_nominal_specify=off  v_out_nominal_value=1  v_out_nominal_unit=V
      settings: InternalSimscapePortConfiguration="{\"Bottom\":[],\"Left\":[{\"id\":\"p_in\",\"label\":\"V+\",\"type\":\"foundation.electrical.electrical\"},{\"id\":\"n_in\",\"label\":\"V-\",\"type\":\"foundation.electrical.electrical\"},{\"id\":\"d\",\"label\":\"d\",\"type\":\"input\"}],\"Right\":[{\"id\":\"p_out\",\"label\":\"Vo+\",\"type\":\"foundation.electrical.electrical\"},{\"id\":\"n_out\",\"label\":\"Vo-\",\"type\":\"foundation.electrical.electrical\"}],\"Top\":[]}"
  DAB Generalized Average Model1 : datacenter_lib/DAB Generalized Average Model  N=5.5  L1=3.4e-05 H  L2=1.12e-06 H  Rt=0.005 Ohm  Co=0.001 F  fs=20000 Hz  vo0_init=800 V  it1R_init=0 A  it1I_init=0 A  include_esr=false  Rc=0.25 Ohm  i_in_specify=on  i_in_priority=None  i_in=0 A  i_in_nominal_specify=off  i_in_nominal_value=1  i_in_nominal_unit=A  i_out_specify=on  i_out_priority=None  i_out=0 A  i_out_nominal_specify=off  i_out_nominal_value=1  i_out_nominal_unit=A  v_in_specify=on  v_in_priority=None  v_in=0 V  v_in_nominal_specify=off  v_in_nominal_value=1  v_in_nominal_unit=V  v_out_specify=on  v_out_priority=None  v_out=0 V  v_out_nominal_specify=off  v_out_nominal_value=1  v_out_nominal_unit=V
      settings: InternalSimscapePortConfiguration="{\"Bottom\":[],\"Left\":[{\"id\":\"p_in\",\"label\":\"V+\",\"type\":\"foundation.electrical.electrical\"},{\"id\":\"n_in\",\"label\":\"V-\",\"type\":\"foundation.electrical.electrical\"},{\"id\":\"d\",\"label\":\"d\",\"type\":\"input\"}],\"Right\":[{\"id\":\"p_out\",\"label\":\"Vo+\",\"type\":\"foundation.electrical.electrical\"},{\"id\":\"n_out\",\"label\":\"Vo-\",\"type\":\"foundation.electrical.electrical\"}],\"Top\":[]}"
  DAB Generalized Average Model2 : datacenter_lib/DAB Generalized Average Model  N=5.5  L1=3.4e-05 H  L2=1.12e-06 H  Rt=0.005 Ohm  Co=0.001 F  fs=20000 Hz  vo0_init=800 V  it1R_init=0 A  it1I_init=0 A  include_esr=false  Rc=0.25 Ohm  i_in_specify=on  i_in_priority=None  i_in=0 A  i_in_nominal_specify=off  i_in_nominal_value=1  i_in_nominal_unit=A  i_out_specify=on  i_out_priority=None  i_out=0 A  i_out_nominal_specify=off  i_out_nominal_value=1  i_out_nominal_unit=A  v_in_specify=on  v_in_priority=None  v_in=0 V  v_in_nominal_specify=off  v_in_nominal_value=1  v_in_nominal_unit=V  v_out_specify=on  v_out_priority=None  v_out=0 V  v_out_nominal_specify=off  v_out_nominal_value=1  v_out_nominal_unit=V
      settings: InternalSimscapePortConfiguration="{\"Bottom\":[],\"Left\":[{\"id\":\"p_in\",\"label\":\"V+\",\"type\":\"foundation.electrical.electrical\"},{\"id\":\"n_in\",\"label\":\"V-\",\"type\":\"foundation.electrical.electrical\"},{\"id\":\"d\",\"label\":\"d\",\"type\":\"input\"}],\"Right\":[{\"id\":\"p_out\",\"label\":\"Vo+\",\"type\":\"foundation.electrical.electrical\"},{\"id\":\"n_out\",\"label\":\"Vo-\",\"type\":\"foundation.electrical.electrical\"}],\"Top\":[]}"
  Delay : Delay  DelayLength=1
  Delay1 : Delay  DelayLength=1  InitialCondition=1
  Electrical Reference : fl_lib/Electrical/Electrical Elements/Electrical Reference
  Gain : Gain  Gain=1/dcOutputVoltage
  Low-Pass Filter (Discrete or Continuous) : eeGeneralControl/Low-Pass Filter (Discrete or Continuous)  K=1  T=0.005  B=inf  A=-inf  init_option=Inherited from block input  x0=0  Ts=-1
  PS-Simulink Converter : nesl_utility/PS-Simulink Converter  PhysicalDomain=network_engine_domain  SubClassName=ps_output  LeftPortType=input  RightPortType=output  PseudoPeriodic=off  Frequencies=[]  VectorFormat=inherit  Unit=inherit  AffineConversion=off
  PS-Simulink Converter1 : nesl_utility/PS-Simulink Converter  PhysicalDomain=network_engine_domain  SubClassName=ps_output  LeftPortType=input  RightPortType=output  PseudoPeriodic=off  Frequencies=[]  VectorFormat=inherit  Unit=inherit  AffineConversion=off
  Simulink-PS Converter : nesl_utility/Simulink-PS Converter  PhysicalDomain=network_engine_domain  SubClassName=ps_input  LeftPortType=input  RightPortType=output  PseudoPeriodic=off  Frequencies=[]  NoiseDistribution=none  NoiseParameters=[]  Unit=1  AffineConversion=off  FilteringAndDerivatives=provide  SimscapeFilterOrder=1  InputFilterTimeConstant=0.001  UdotUserProvided=0
  Simulink-PS Converter1 : nesl_utility/Simulink-PS Converter  PhysicalDomain=network_engine_domain  SubClassName=ps_input  LeftPortType=input  RightPortType=output  PseudoPeriodic=off  Frequencies=[]  NoiseDistribution=none  NoiseParameters=[]  Unit=1  AffineConversion=off  FilteringAndDerivatives=provide  SimscapeFilterOrder=1  InputFilterTimeConstant=0.001  UdotUserProvided=0
  Voltage Sensor : fl_lib/Electrical/Electrical Sensors/Voltage Sensor
  Voltage Sensor1 : fl_lib/Electrical/Electrical Sensors/Voltage Sensor
  AC + : PMIOPort  Side=Left
  AC - : PMIOPort  Port=2  Side=Left
  + : PMIOPort  Port=3  Side=Right
  - : PMIOPort  Port=4  Side=Right
  Out1 : Outport
  V_out_pu : Outport  Port=2
  wires:
  ma/1 -> Simulink-PS Converter1/1
  Gain/1 -> V_out_pu/1
  PhA/1 -> Simulink-PS Converter/1
  Delay1/1 -> Gain/1
  PS-Simulink Converter1/1 -> Delay1/1
  Low-Pass Filter (Discrete or Continuous)/1 -> Out1/1
  Delay/1 -> Low-Pass Filter (Discrete or Continuous)/1
  PS-Simulink Converter/1 -> Delay/1
  connections:
  Simulink-PS Converter1/RConn1 -- CHB Phase Leg (Average Model)/LConn3
  Array Connection1/RConn1 -- CHB Phase Leg (Average Model)/RConn2
  Array Connection/RConn1 -- CHB Phase Leg (Average Model)/RConn1
  DAB Generalized Average Model/LConn3 -- DAB Generalized Average Model1/LConn3 -- DAB Generalized Average Model2/LConn3 -- Simulink-PS Converter/RConn1
  PS-Simulink Converter1/LConn1 -- Voltage Sensor1/RConn1
  DAB Generalized Average Model1/RConn2 -- DAB Generalized Average Model2/RConn2 -- DAB Generalized Average Model/RConn2 -- Voltage Sensor1/RConn2 -- Electrical Reference/LConn1 -- -/RConn1
  DAB Generalized Average Model/RConn1 -- DAB Generalized Average Model1/RConn1 -- DAB Generalized Average Model2/RConn1 -- Voltage Sensor1/LConn1 -- +/RConn1
  DAB Generalized Average Model/LConn2 -- Array Connection1/LConn1 -- Capacitor/RConn1 -- Voltage Sensor/RConn2
  CHB Phase Leg (Average Model)/LConn2 -- AC -/RConn1
  Capacitor2/LConn1 -- Array Connection/LConn3 -- DAB Generalized Average Model2/LConn1
  Capacitor2/RConn1 -- Array Connection1/LConn3 -- DAB Generalized Average Model2/LConn2
  CHB Phase Leg (Average Model)/LConn1 -- AC +/RConn1
  DAB Generalized Average Model/LConn1 -- Capacitor/LConn1 -- Array Connection/LConn1 -- Voltage Sensor/LConn1
  Capacitor1/RConn1 -- Array Connection1/LConn2 -- DAB Generalized Average Model1/LConn2
  Capacitor1/LConn1 -- Array Connection/LConn2 -- DAB Generalized Average Model1/LConn1
  PS-Simulink Converter/LConn1 -- Voltage Sensor/RConn1
